simulink model "robertoWRosTestedIssues"  (R2018a)
settings: Solver=VariableStepAuto  StartTime=0.0  StopTime=200  RelTol=1e-3
InitFcn:
  | load('joystick_ref_002.mat')
  | 
  | %Vehicle Lead gains
  | a2=26.4941;
  | b2=0.2667;
  | K2=80.4;
  | 
  | % T = 20;
  | a = 5;
  | b = 0.4;
  | 
  | % PID Gains
  | kp = 0.1;
  | %kp = 2*b/a^2;
  | 
  | % DAS
  | DT=2;
  | gamma1sq=0.2;
  | gamma2sq=0.1;
  | 
  | 
  | %initSub = rossubscriber('/ship/state');
  | %initMsg = receive(initSub,10)
  | 
  | %y_ref=initMsg.Pose.X
  | 
  | y_ref=0;
libraries: simulink x8, robotlib x2, vrlib x1, realtime_pacer_lib x1
settings Model: SimulationMode=accelerator  Creator=transmogrifier  LastModifiedBy=transmogrifier

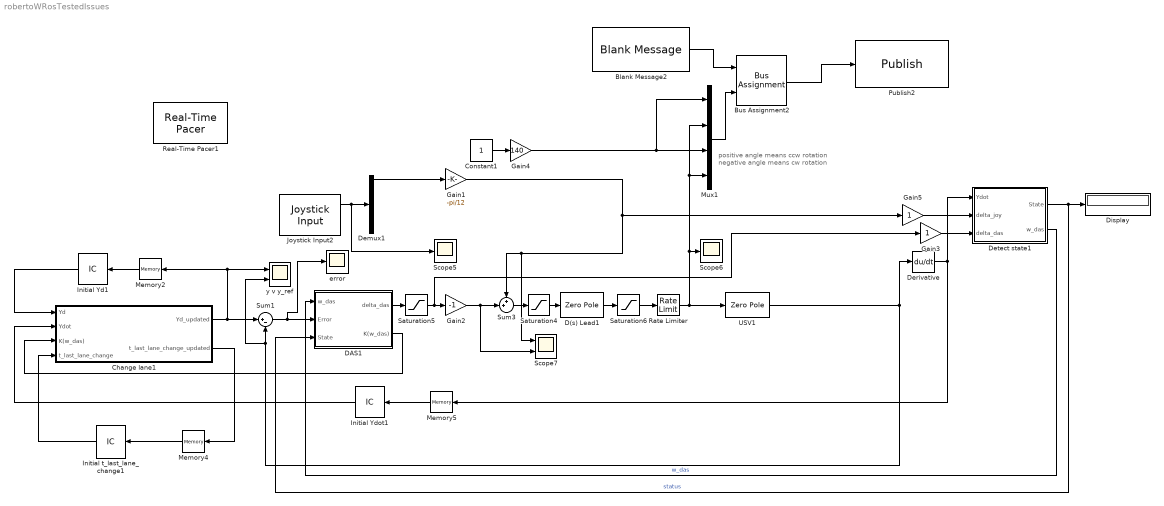
== system robertoWRosTestedIssues ==
  note: positive angle means ccw rotation
      | negative angle means cw rotation
  Blank Message2 : robotlib/Blank Message  SourceLibraryInfo=This block requires Robotics System Toolbox  messageType=usv16_msgs/Usv16ActuatorInputs  SampleTime=inf
      settings: SourceProductBaseCode=RO
  Bus Assignment2 : BusAssignment  AssignedSignals=ActuatorInputs
  Change lane1 : Subsystem
  Constant1 : Constant
  D(s) Lead1 : ZeroPole  Zeros=[-b2]  Poles=[-a2]  Gain=[K2]
  DAS1 : Subsystem
  Demux1 : Demux  Outputs=8
  Derivative : Derivative
  Detect state1 : Subsystem
  Display : Display
  Gain1 : Gain  Gain=-pi/12
  Gain2 : Gain  Gain=-1
  Gain3 : Gain
  Gain4 : Gain  Gain=140
  Gain5 : Gain
  Initial Yd1 : InitialCondition  Value=y_ref
  Initial Ydot1 : InitialCondition  Value=0
  Initial t_last_lane_change1 : InitialCondition  Value=0
  Joystick Input2 : vrlib/Joystick Input  joyid=1  adjustports=on  forcefeed=off
      settings: SourceProductBaseCode=VR
  Memory2 : Memory
  Memory4 : Memory
  Memory5 : Memory
  Mux1 : Mux
  Publish2 : robotlib/Publish  SourceLibraryInfo=This block requires Robotics System Toolbox  topicSource=Select from ROS network  topic=/ship/actuation  messageType=usv16_msgs/Usv16ActuatorInputs  messageQueueLength=1
      settings: SourceProductBaseCode=RO
  Rate Limiter : RateLimiter  RisingSlewLimit=0.5  FallingSlewLimit=-0.5  SampleTimeMode=inherited
  Real-Time Pacer1 : realtime_pacer_lib/Real-Time Pacer  simTimePerRealTime=1
  Saturation4 : Saturate  UpperLimit=pi/12  LowerLimit=-pi/12
  Saturation5 : Saturate  UpperLimit=pi/12  LowerLimit=-pi/12
  Saturation6 : Saturate  UpperLimit=pi/12  LowerLimit=-pi/12
  Scope5 : Scope
  Scope6 : Scope
  Scope7 : Scope  NumInputPorts=2
  Sum1 : Sum  Inputs=|+-
  Sum3 : Sum  Inputs=++|
  USV1 : ZeroPole  Zeros=[]  Poles=[0 0 -3]  Gain=[2]
  error : Scope
  y v y_ref : Scope  NumInputPorts=2
  wires:
  Initial t_last_lane_change1/1 -> Change lane1/4(t_last_lane_change)
  Initial Ydot1/1 -> Change lane1/2(Ydot)
  Initial Yd1/1 -> Change lane1/1(Yd)
  D(s) Lead1/1 -> Saturation6/1
  Change lane1/2(t_last_lane_change_updated) -> Memory4/1
  Memory5/1 -> Initial Ydot1/1
  Memory4/1 -> Initial t_last_lane_change1/1
  Memory2/1 -> Initial Yd1/1
  Sum1/1 -> error/1, DAS1/2(Error)
  Saturation4/1 -> D(s) Lead1/1
  Demux1/1 -> Gain1/1
  USV1/1 -> Derivative/1, y v y_ref/2, Sum1/2
  Change lane1/1(Yd_updated) -> Memory2/1, y v y_ref/1, Sum1/1
  Joystick Input2/1 -> Scope5/1, Demux1/1
  DAS1/2(K(w_das)) -> Change lane1/3(K(w_das))
  Sum3/1 -> Saturation4/1
  Detect state1/1(State) -> Display/1, DAS1/3(State)  "status"
  Detect state1/2(w_das) -> DAS1/1(w_das)  "w_das"
  Blank Message2/1 -> Bus Assignment2/1
  Saturation6/1 -> Rate Limiter/1
  Mux1/1 -> Bus Assignment2/2
  Gain4/1 -> Mux1/1, Mux1/3
  Bus Assignment2/1 -> Publish2/1
  Constant1/1 -> Gain4/1
  DAS1/1(delta_das) -> Saturation5/1
  Rate Limiter/1 -> USV1/1, Scope6/1, Mux1/4, Mux1/2
  Gain1/1 -> Gain5/1, Scope7/1, Sum3/1
  Saturation5/1 -> Gain3/1, Gain2/1
  Gain5/1 -> Detect state1/2(delta_joy)
  Gain3/1 -> Detect state1/3(delta_das)
  Derivative/1 -> Memory5/1, Detect state1/1(Ydot)
  Gain2/1 -> Scope7/2, Sum3/2

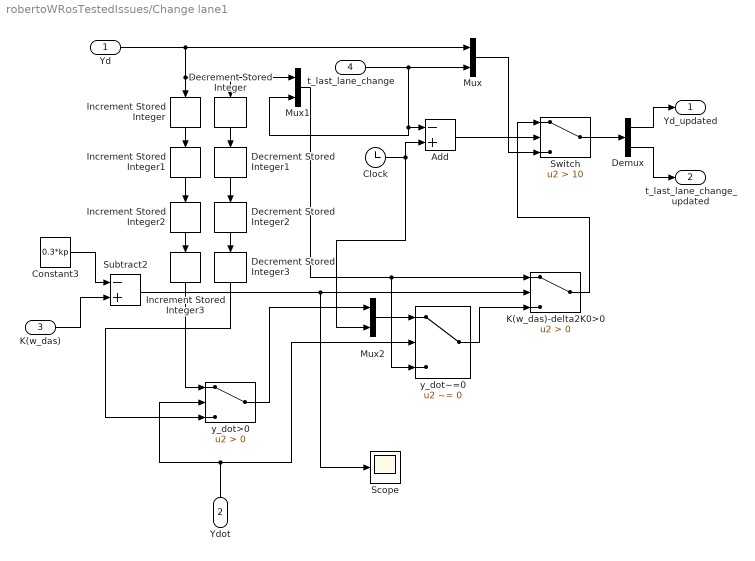
== system robertoWRosTestedIssues/Change lane1 ==
  Yd : Inport
  Ydot : Inport  Port=2
  K(w_das) : Inport  Port=3
  t_last_lane_change : Inport  Port=4
  Add : Sum  Inputs=-+
  Clock : Clock
  Constant3 : Constant  Value=0.3*kp
  Decrement Stored Integer{,1..3} (4 alike) : simulink/Additional Math & Discrete/Additional Math: Increment - Decrement/Decrement Stored Integer
      settings: SourceProductName=Simulink  SourceProductBaseCode=SL
  Demux : Demux  Outputs=2
  Increment Stored Integer{,1..3} (4 alike) : simulink/Additional Math & Discrete/Additional Math: Increment - Decrement/Increment Stored Integer
      settings: SourceProductName=Simulink
  K(w_das)-delta2K0>0 : Switch  Criteria=u2 > Threshold  ZeroCross=off
  Mux : Mux  Inputs=2
  Mux1 : Mux  Inputs=2
  Mux2 : Mux  Inputs=2
  Scope : Scope
  Subtract2 : Sum  Inputs=-+
  Switch : Switch  Criteria=u2 > Threshold  Threshold=10
  y_dot>0 : Switch  Criteria=u2 > Threshold
  y_dot~=0 : Switch  Criteria=u2 ~= 0
  Yd_updated : Outport
  t_last_lane_change_updated : Outport  Port=2
  wires:
  Increment Stored Integer/1 -> Increment Stored Integer1/1
  y_dot>0/1 -> Mux2/1
  K(w_das)/1 -> Subtract2/2
  Yd/1 -> Mux/1, Mux1/1, Decrement Stored Integer/1, Increment Stored Integer/1
  y_dot~=0/1 -> K(w_das)-delta2K0>0/3
  Constant3/1 -> Subtract2/1
  Ydot/1 -> y_dot~=0/2, y_dot>0/2
  Decrement Stored Integer/1 -> Decrement Stored Integer1/1
  Clock/1 -> Mux2/2, Add/2
  t_last_lane_change/1 -> Mux1/2, Add/1, Mux/2
  Add/1 -> Switch/2
  K(w_das)-delta2K0>0/1 -> Switch/1
  Mux/1 -> Switch/3
  Switch/1 -> Demux/1
  Demux/1 -> Yd_updated/1
  Demux/2 -> t_last_lane_change_updated/1
  Mux1/1 -> K(w_das)-delta2K0>0/1, y_dot~=0/3
  Mux2/1 -> y_dot~=0/1
  Subtract2/1 -> Scope/1, K(w_das)-delta2K0>0/2
  Increment Stored Integer1/1 -> Increment Stored Integer2/1
  Increment Stored Integer2/1 -> Increment Stored Integer3/1
  Increment Stored Integer3/1 -> y_dot>0/1
  Decrement Stored Integer1/1 -> Decrement Stored Integer2/1
  Decrement Stored Integer2/1 -> Decrement Stored Integer3/1
  Decrement Stored Integer3/1 -> y_dot>0/3

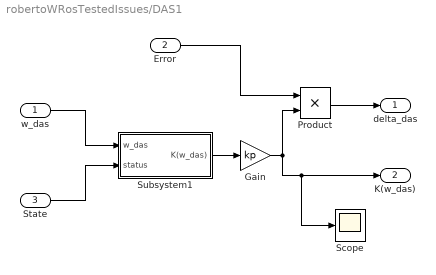
== system robertoWRosTestedIssues/DAS1 ==
  w_das : Inport
  Error : Inport  Port=2
  State : Inport  Port=3
  Gain : Gain  Gain=kp
  Product : Product
  Scope : Scope
  Subsystem1 : Subsystem
  delta_das : Outport
  K(w_das) : Outport  Port=2
  wires:
  Product/1 -> delta_das/1
  Error/1 -> Product/1
  State/1 -> Subsystem1/2(status)
  Subsystem1/1(K(w_das)) -> Gain/1
  Gain/1 -> Product/2, Scope/1, K(w_das)/1
  w_das/1 -> Subsystem1/1(w_das)

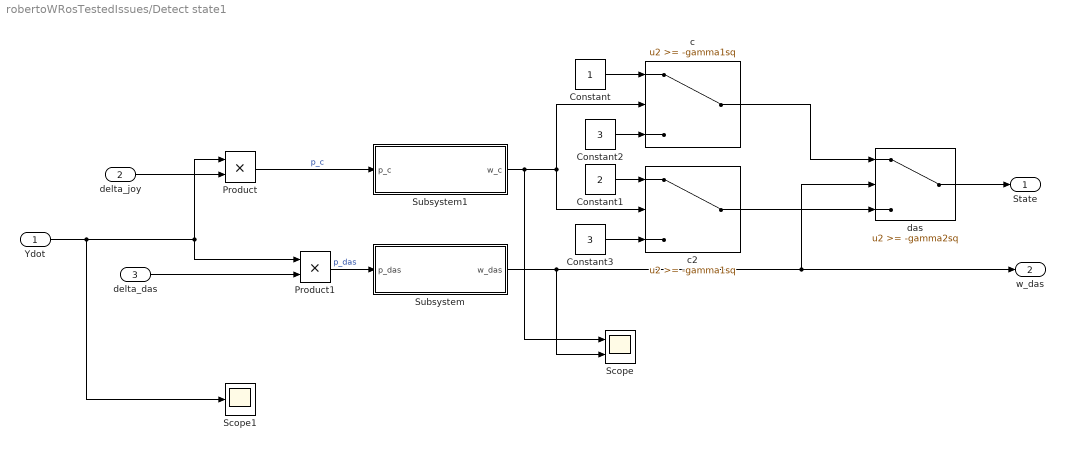
== system robertoWRosTestedIssues/Detect state1 ==
  Ydot : Inport
  delta_joy : Inport  Port=2
  delta_das : Inport  Port=3
  Constant : Constant
  Constant1 : Constant  Value=2
  Constant2 : Constant  Value=3
  Constant3 : Constant  Value=3
  Product : Product
  Product1 : Product
  Scope : Scope  NumInputPorts=2
  Scope1 : Scope
  Subsystem : Subsystem
  Subsystem1 : Subsystem
  c : Switch  Threshold=-gamma1sq
  c2 : Switch  Threshold=-gamma1sq
  das : Switch  Threshold=-gamma2sq
  State : Outport
  w_das : Outport  Port=2
  wires:
  Ydot/1 -> Scope1/1, Product/1, Product1/1
  delta_joy/1 -> Product/2
  delta_das/1 -> Product1/2
  Product/1 -> Subsystem1/1(p_c)  "p_c"
  Product1/1 -> Subsystem/1(p_das)  "p_das"
  Subsystem/1(w_das) -> Scope/2, w_das/1, das/2
  Subsystem1/1(w_c) -> Scope/1, c2/2, c/2
  Constant/1 -> c/1
  c/1 -> das/1
  Constant1/1 -> c2/1
  c2/1 -> das/3
  Constant3/1 -> c2/3
  Constant2/1 -> c/3
  das/1 -> State/1

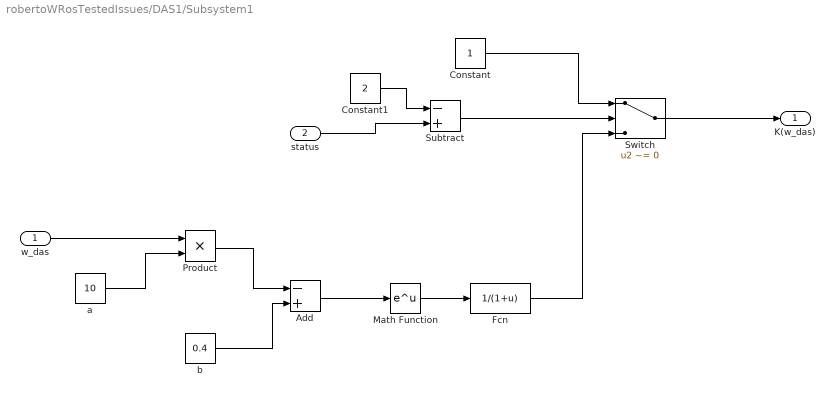
== system robertoWRosTestedIssues/DAS1/Subsystem1 ==
  w_das : Inport
  status : Inport  Port=2
  Add : Sum  Inputs=-+
  Constant : Constant
  Constant1 : Constant  Value=2
  Fcn : Fcn  Expr=1/(1+u)
  Math Function : Math  SaturateOnIntegerOverflow=on
  Product : Product
  Subtract : Sum  Inputs=-+
  Switch : Switch  Criteria=u2 ~= 0
  a : Constant  Value=10
  b : Constant  Value=0.4
  K(w_das) : Outport
  wires:
  w_das/1 -> Product/1
  a/1 -> Product/2
  Product/1 -> Add/1
  b/1 -> Add/2
  Add/1 -> Math Function/1
  Math Function/1 -> Fcn/1
  Fcn/1 -> Switch/3
  Constant/1 -> Switch/1
  Switch/1 -> K(w_das)/1
  Constant1/1 -> Subtract/1
  status/1 -> Subtract/2
  Subtract/1 -> Switch/2

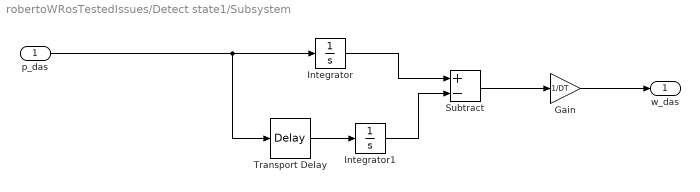
== system robertoWRosTestedIssues/Detect state1/Subsystem ==
  p_das : Inport
  Gain : Gain  Gain=1/DT
  Integrator : Integrator
  Integrator1 : Integrator
  Subtract : Sum  Inputs=+-
  Transport Delay : TransportDelay  DelayTime=DT
  w_das : Outport
  wires:
  Subtract/1 -> Gain/1
  Gain/1 -> w_das/1
  Transport Delay/1 -> Integrator1/1
  Integrator1/1 -> Subtract/2
  Integrator/1 -> Subtract/1
  p_das/1 -> Transport Delay/1, Integrator/1

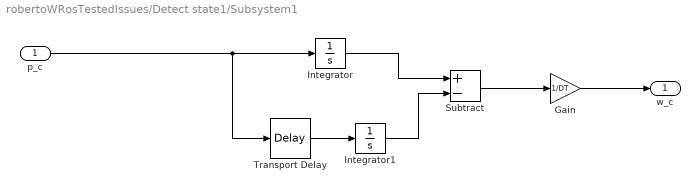
== system robertoWRosTestedIssues/Detect state1/Subsystem1 ==
  p_c : Inport
  Gain : Gain  Gain=1/DT
  Integrator : Integrator
  Integrator1 : Integrator
  Subtract : Sum  Inputs=+-
  Transport Delay : TransportDelay  DelayTime=DT
  w_c : Outport
  wires:
  p_c/1 -> Integrator/1, Transport Delay/1
  Integrator/1 -> Subtract/1
  Integrator1/1 -> Subtract/2
  Transport Delay/1 -> Integrator1/1
  Gain/1 -> w_c/1
  Subtract/1 -> Gain/1
